simulink model "sl_synch"  (Simulink 7.4)
settings: Solver=VariableStepDiscrete  StartTime=0.0  StopTime=inf  MaxStep=.01  RelTol=1e-3
PostLoadFcn:
  | % Load the GUI
  | h_synch_gui = sl_synch_gui;
  | 
  | % Adjust its position
  | set(h_synch_gui,'Position',[74.4 28 63 18.08])
StartFcn:
  | % The user may have closed the GUI
  | try
  | 
  | % Get the string of the startstop pushbutton.
  | mystring = get(findobj(h_synch_gui,'Tag','pushbutton_startstop'),'String');
  | 
  | % See if the string is "Start Simulation."
  | % If it is, that implies that the start wasn't driven by the GUI.
  | % Thus we need to update the GUI by making a callback to the startstop function.
  | if strcmp(mystring,'Start Simulation')
  |   sl_synch_gui('pushbutton_startstop_Callback',startstop_hObject,[],sl_synch_handles)
  | end
  | 
  | end
StopFcn:
  | % The user may have closed the GUI
  | try
  | 
  | % Get the string of the startstop pushbutton.
  | mystring = get(findobj(h_synch_gui,'Tag','pushbutton_startstop'),'String');
  | 
  | % See if the string is "Stop Simulation."
  | % If it is, that implies that the stop wasn't driven by the GUI.
  | % Thus we need to update the GUI by making a callback to the startstop function.
  | if strcmp(mystring,'Stop Simulation')
  |   sl_synch_gui('pushbutton_startstop_Callback',startstop_hObject,[],sl_synch_handles)
  | end
  | 
  | end
CloseFcn:
  | % Try to close the GUI
  | % The user might have already closed it.
  | try
  |   close(h_synch_gui)
  | end
settings Model: Creator=wcampbel  LastModifiedBy=wcampbel
settings DebuggingCC: StrictBusMsg=ErrorLevel1

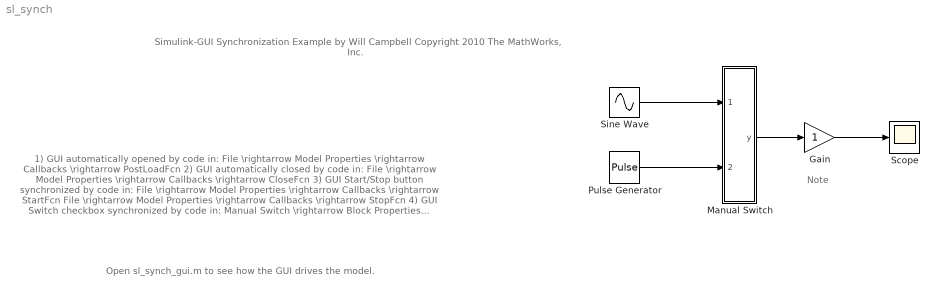
== system sl_synch ==
  note: Simulink-GUI Synchronization Example
      | by Will Campbell
      | Copyright 2010 The MathWorks, Inc.
  note: 1) GUI automatically opened by code in:
      |      File \rightarrow Model Properties \rightarrow Callbacks \rightarrow PostLoadFcn
      | 2) GUI automatically closed by code in:
      |      File \rightarrow Model Properties \rightarrow Callbacks \rightarrow CloseFcn
      | 3) GUI Start/Stop button synchronized by code in:
      |      File \rightarrow Model Properties \rightarrow Callbacks \rightarrow StartFcn
      |      File \rightarrow Model Properties \rightarrow Callbacks \rightarrow StopFcn
      | 4) GUI Switch checkbox synchronized by code in:
      |      Manual Switch \rightarrow Block Properties \rightarrow Callbacks \rightarrow OpenFcn
  note: Open sl_synch_gui.m to see how the GUI drives the model.
  note: Note
  Gain : Gain  ParameterDataType=fixdt(1, 16)  ParameterScaling=2^0  OutDataType=fixdt(1, 16)  OutScaling=2^0
  Manual Switch : Subsystem  StopFcn=manswitch_config stop;  mask(Manual Switch){sw=1, action=0, varsize=off}
      mask prompts: sw "Current setting:"; varsize "Allow different input sizes (Results in variable-size output signal)"
      mask help: Output toggles between two inputs by double-clicking on the block.
      mask init:
      | x=1; y=1;
      | [x,y]=manswitch;
      | manswitch_config;
      settings: ErrorFcn=manswitch
      settings: OpenFcn=|
      | manswitch Open;
      | 
      | % This portion synchs the switch to the GUI
      | try
      | % Get the value of the switch checkbox.
      | myvalue = get(findobj(h_synch_gui,'Tag','checkbox_switch'),'Value');
      | 
      | % Reassign the value
      | set(findobj(h_synch_gui,'Tag','checkbox_switch'),'Value',abs(myvalue-1))
      | 
      | end
      mask Help: This block implements a manual switch.
      mask Display: plot(x,y)
  Pulse Generator : DiscretePulseGenerator  PulseType=Time based  Amplitude=1  Period=2.5  PulseWidth=25  PhaseDelay=3  SampleTime=1
  Scope : Scope
      settings: TimeRange=10  YMin=-10  YMax=10
  Sine Wave : Sin  Amplitude=1  Bias=0  Frequency=1  Phase=0  Samples=10  SampleTime=0  Offset=0
  wires:
  Pulse Generator/1 -> Manual Switch/2(u2)
  Sine Wave/1 -> Manual Switch/1(u1)
  Manual Switch/1(y) -> Gain/1
  Gain/1 -> Scope/1

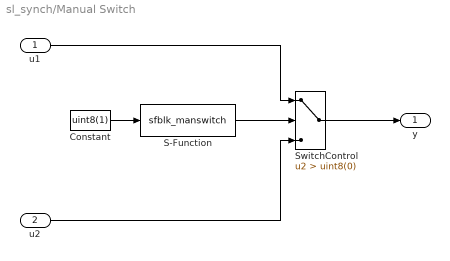
== system sl_synch/Manual Switch ==
  u1 : Inport  OutDataType=fixdt(1, 16)  OutScaling=2^0
  u2 : Inport  Port=2  OutDataType=fixdt(1, 16)  OutScaling=2^0
  Constant : Constant  DisableCoverage=on  Value=uint8(1)  OutDataType=fixdt(1, 16)  OutScaling=2^0
  S-Function : S-Function  DisableCoverage=on  FunctionName=sfblk_manswitch  EnableBusSupport=off
  SwitchControl : Switch  Criteria=u2 > Threshold  Threshold=uint8(0)  OutDataType=fixdt(1, 16)  OutScaling=2^0
  y : Outport  OutDataType=fixdt(1, 16)  OutScaling=2^0
  wires:
  Constant/1 -> S-Function/1
  S-Function/1 -> SwitchControl/2
  u1/1 -> SwitchControl/1
  u2/1 -> SwitchControl/3
  SwitchControl/1 -> y/1
